simulink model "HR"  (R2022a)
settings: Solver=FixedStepDiscrete  StartTime=0.0  StopTime=0.04  FixedStep=0.04  RelTol=1e-3
PreLoadFcn:
  | listing = dir;
  | if (contains([listing .name], 'AGR')) && (contains([listing .name], 'MAP'))
  |     addpath('./AGR', './MAP');
  |     addpath( genpath('./MAP') );
  | elseif (contains([listing .name], 'HR.slx'))
  |     addpath('../AGR', '../MAP');
  |     addpath( genpath('../MAP') );
  | else
  | 
  | end
  | 
  | load('BusStructureHR.mat');
InitFcn:
  | listing = dir;
  | if (contains([listing .name], 'AGR')) && (contains([listing .name], 'MAP'))
  |     addpath('./AGR', './MAP');
  |     addpath( genpath('./MAP') );
  | elseif (contains([listing .name], 'HR.slx'))
  |     addpath('../AGR', '../MAP');
  |     addpath( genpath('../MAP') );
  | else
  | 
  | end
  | 
  | load('BusStructureHR.mat');
StartFcn:
  | listing = dir;
  | if (contains([listing .name], 'AGR')) && (contains([listing .name], 'MAP'))
  |     addpath('./AGR', './MAP');
  |     addpath( genpath('./MAP') );
  | elseif (contains([listing .name], 'HR.slx'))
  |     addpath('../AGR', '../MAP');
  |     addpath( genpath('../MAP') );
  | else
  | 
  | end
  | 
  | load('BusStructureHR.mat');
undefined symbols (not defined in the file or in its folder): HRDataTagWrap, HRElevationValid, HRImpactPointElevation, HRSelected, HRSelectedWraparound, HRTargetOffMap, HRTargetRangeEast, HRTargetRangeNorth, isFeasible, llh, ne, ned2ECEF, pECEF_ip, pECEF_ref, statusCode, targetLLH, targetNE
libraries: aerolibconvert2 x1
settings Model: Creator=ASCL  LastModifiedBy=ASCL
settings DataIOCC: SaveOutput=off  SignalLogging=off  DSMLogging=off  SaveTime=off  ReturnWorkspaceOutputs=off
settings OptimizationCC: BlockReduction=off  DefaultParameterBehavior=Inlined  UseDivisionForNetSlopeComputation=on  GainParamInheritBuiltInType=on  UseFloatMulNetSlope=on  ExpressionFolding=off  PassReuseOutputArgsAs=Individual arguments  ZeroExternalMemoryAtStartup=off  ZeroInternalMemoryAtStartup=off  EfficientFloat2IntCast=on  LifeSpan=inf  OptimizeBlockOrder=speed  DifferentSizesBufferReuse=on  EfficientTunableParamExpr=on
settings DebuggingCC: SignalInfNanChecking=warning  ReadBeforeWriteMsg=EnableAllAsWarning  WriteAfterWriteMsg=EnableAllAsError  WriteAfterReadMsg=EnableAllAsError  IntegerOverflowMsg=error  ParameterTunabilityLossMsg=error  UniqueDataStoreMsg=error  AssertControl=DisableAll  NonBusSignalsTreatedAsBus=error  SFInvalidInputDataAccessInChartInitDiag=error  SFTransitionOutsideNaturalParentDiag=error  SFUnreachableExecutionPathDiag=error  SFUndirectedBroadcastEventsDiag=error  IntegerSaturationMsg=error
settings HardwareCC: ProdBitPerPointer=32  ProdBitPerSizeT=32  ProdBitPerPtrDiffT=32  ProdLargestAtomicInteger=Long  ProdLargestAtomicFloat=Double  ProdEndianess=BigEndian  ProdWordSize=32  ProdLongLongMode=on  ProdHWDeviceType=Freescale->MPC83xx
settings ModelReferenceCC: ModelReferenceNumInstancesAllowed=Single
settings SFSimCC: SimCustomHeaderCode="#include \"MAP.h\""  SimUserSources=MAP.c  SimUserLibraries=WS2_32.LIB  CompileTimeRecursionLimit=0  EnableRuntimeRecursion=off  MATLABDynamicMemAlloc=off
settings RTWCC: SystemTargetFile=ert.tlc  TemplateMakefile=ert_default_tmf  GenerateReport=on  RTWUseSimCustomCode=on  CustomHeaderCode="#include \"MAP.h\""  CustomSource=MAP.c  CustomLibrary=WS2_32.LIB  BuildConfiguration=Faster Runs  IncludeHyperlinkInReport=on  LaunchReport=on  GenerateTraceInfo=on  GenerateTraceReport=on  GenerateTraceReportSl=on  GenerateTraceReportSf=on  GenerateTraceReportEml=on  GenerateCodeMetricsReport=on
settings CodeAppCC: ForceParamTrailComments=on  IgnoreCustomStorageClasses=off  OperatorAnnotations=on  SimulinkDataObjDesc=on  SFDataObjDesc=on  MATLABFcnDesc=on  InsertBlockDesc=on  StateflowObjectComments=on  MATLABSourceComments=on  EnableCustomComments=on  InlinedPrmAccess=Macros  ReqsInCode=on
settings ERTTargetCC: TargetLangStandard=C99 (ISO)  UtilityFuncGeneration=Shared location  GenerateSampleERTMain=on  IncludeMdlTerminateFcn=off  CombineSignalStateStructs=on  SuppressErrorStatus=on  SupportAbsoluteTime=off  SupportNonFinite=off  SupportComplex=off  SupportVariableSizeSignals=on  ParenthesesLevel=Standards  CastingMode=Standards  GenerateSharedConstants=off  InlinedParameterPlacement=NonHierarchical  ERTCustomFileTemplate=example_file_process.tlc  RateTransitionBlockCode=Function  PreserveIfCondition=on  ConvertIfToSwitch=off  EnableSignedLeftShifts=off  EnableSignedRightShifts=off

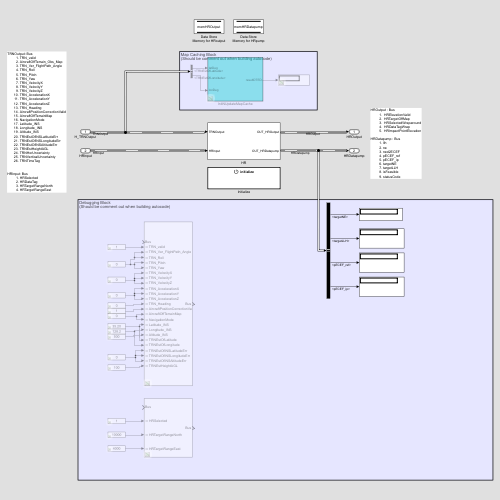
[thumbnail: Simulink's stored preview of the top-level diagram]
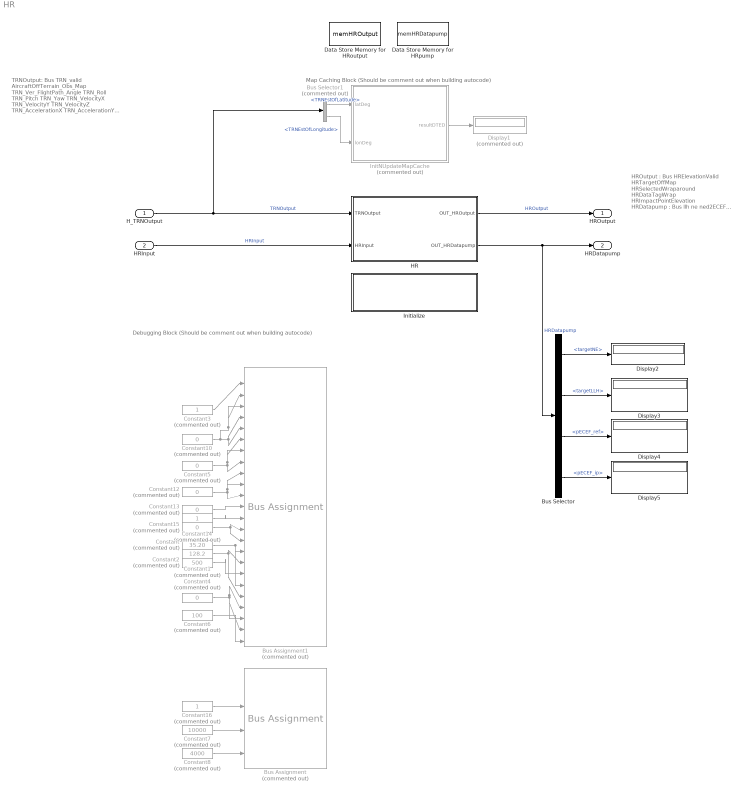
== system HR ==
  note: Debugging Block
      | (Should be comment out when building autocode)
  note: TRNOutput: Bus
      | TRN_valid
      | AircraftOffTerrain_Obs_Map
      | TRN_Ver_FlightPath_Angle
      | TRN_Roll
      | TRN_Pitch
      | TRN_Yaw
      | TRN_VelocityX
      | TRN_VelocityY
      | TRN_VelocityZ
      | TRN_AccelerationX
      | TRN_AccelerationY
      | TRN_AccelerationZ
      | TRN_Heading
      | AircraftPositionCorrectionValid
      | AircraftOffTerrainMap
      | NavigationMode
      | Latitude_INS
      | Longitude_INS
      | Altitude_INS
      | TRNEstOfINSLatitudeErr
      | TRNEstOfINSLongitudeErr
      | TRNEstOfINSAltitudeErr
      | TRNEstHeightAGL
      | TRNHorUncertainty
      | TRNVerticalUncertainty
      | TRNTimeTag
      |
      | HRInput: Bus
      | HRSelected
      | HRDataTag
      | HRTargetRangeNorth
      | HRTargetRangeEast
  note: HROutput : Bus
      | HRElevationValid
      | HRTargetOffMap
      | HRSelectedWraparound
      | HRDataTagWrap
      | HRImpactPointElevation
      |
      | HRDatapump : Bus
      | llh
      | ne
      | ned2ECEF
      | pECEF_ref
      | pECEF_ip
      | targetNE
      | targetLLH
      | isFeasible
      | statusCode
  note: Map Caching Block
      | (Should be comment out when building autocode)
  H_TRNOutput : Inport  OutDataTypeStr=Bus: TRNOutput  Interpolate=off  BusOutputAsStruct=on
  HRInput : Inport  Port=2  OutDataTypeStr=Bus: HRInput  Interpolate=off  BusOutputAsStruct=on
  Bus Assignment : BusAssignment  Commented=on  AssignedSignals=HRSelected,HRTargetRangeNorth,HRTargetRangeEast
  Bus Assignment1 : BusAssignment  Commented=on  AssignedSignals=TRN_valid,TRN_Ver_FlightPath_Angle,TRN_Roll,TRN_Pitch,TRN_Yaw,TRN_VelocityX,TRN_VelocityY,TRN_VelocityZ,TRN_AccelerationX,TRN_AccelerationY,TRN_AccelerationZ,TRN_Heading,AircraftPositionCorrectionValid,AircraftOffTerrainMap,NavigationMode,Latitude_INS,Longitude_INS,Altitude_INS,TRNEstOfLatitude,TRNEstOfLongitude,TRNEstOfINSLatitudeErr,TRNEstOfINSLongitudeErr,TRNEstOfINSAltitudeErr,TRNEstHeightAGL
  Bus Selector : BusSelector  OutputSignals=targetNE,targetLLH,pECEF_ref,pECEF_ip
  Bus Selector1 : BusSelector  Commented=on  OutputSignals=TRNEstOfLatitude,TRNEstOfLongitude
  Constant : Constant  Commented=on  Value=35.20
  Constant1 : Constant  Commented=on  Value=128.2
  Constant{4..5,10,12..13} (5 alike) : Constant  Commented=on  Value=0
  Constant14 : Constant  Commented=on  OutDataTypeStr=boolean
  Constant15 : Constant  Commented=on  Value=0  OutDataTypeStr=boolean
  Constant16 : Constant  Commented=on  OutDataTypeStr=boolean
  Constant2 : Constant  Commented=on  Value=500
  Constant3 : Constant  Commented=on  OutDataTypeStr=boolean
  Constant6 : Constant  Commented=on  Value=100  OutDataTypeStr=uint16
  Constant7 : Constant  Commented=on  Value=10000  OutDataTypeStr=double
  Constant8 : Constant  Commented=on  Value=4000  OutDataTypeStr=double
  Data Store Memory for HRoutput : DataStoreMemory  DataStoreName=memHROutput  ReadBeforeWriteMsg=warning  WriteAfterWriteMsg=warning  WriteAfterReadMsg=warning  VectorParams1D=off  ShowAdditionalParam=off  OutDataTypeStr=Bus: HROutput
  Data Store Memory for HRpump : DataStoreMemory  DataStoreName=memHRDatapump  ReadBeforeWriteMsg=warning  WriteAfterWriteMsg=warning  WriteAfterReadMsg=warning  VectorParams1D=off  ShowAdditionalParam=off  OutDataTypeStr=Bus: HRDatapump
  Display1 : Display  Commented=on
  Display{2..5} (4 alike) : Display
  HR : Subsystem
      mask init:
      | % latGPS = double(0);
      | % lonGPS = double(0);
      | % altGPS = double(0);
      | % velEGPS = double(0);
      | % velNGPS = double(0);
      | % velUGPS = double(0);
      | % notValidGPS = boolean(0);
      | % notAvaildINS = boolean(0);
      | % velUINS = double(0);
      | % velVINS = double(0);
      | % velWINS = double(0);
      | % rollINS = double(0);
      | % pitchINS = double(0);
      | % hgdINS = double(0);
      | % accXINS = double(0);
      | % accYINS = double(0);
      | % accZINS = double(0);
      | % activated = boolean(0);
      | % reactionT = uint16(0);
      | % pullUpG = uint16(0);
      | % rollRate = uint16(0);
      | % gOnsetRate = uint16(0);
      | % maxGamma = uint16(0);
      | % setWarnH = double(0);
      | % obsWarningTime = uint16(1);
      | % wiresWarningTime = uint16(1);
      | % latErrOfINS = double(0);
      | % lonErrOfINS = double(0);
      | % altErrorofINS = uint16(0);
      | % heightEstOfTRN = uint16(0);
      | % horUncertaintyOfTRN = double(0);
      | % verUncertaintyOfTRN = double(0);
  InitNUpdateMapCache : Subsystem  Commented=on  TreatAsAtomicUnit=on
  Initialize : Subsystem  TreatAsAtomicUnit=on
  HROutput : Outport  OutDataTypeStr=Bus: HROutput  VectorParamsAs1DForOutWhenUnconnected=off  BusOutputAsStruct=on
  HRDatapump : Outport  Port=2  OutDataTypeStr=Bus: HRDatapump  VectorParamsAs1DForOutWhenUnconnected=off  BusOutputAsStruct=on
  wires:
  Constant8/1 -> Bus Assignment/4
  Bus Selector/4 -> Display5/1  "<pECEF_ip>"
  Bus Selector/2 -> Display3/1  "<targetLLH>"
  H_TRNOutput/1 -> Bus Selector1/1, HR/1(TRNOutput)  "TRNOutput"
  Bus Selector/3 -> Display4/1  "<pECEF_ref>"
  Constant5/1 -> Bus Assignment1/7, Bus Assignment1/8, Bus Assignment1/9
  Constant6/1 -> Bus Assignment1/25
  Constant12/1 -> Bus Assignment1/10, Bus Assignment1/11, Bus Assignment1/12
  HRInput/1 -> HR/2(HRInput)  "HRInput"
  HR/2(OUT_HRDatapump) -> Bus Selector/1, HRDatapump/1  "HRDatapump"
  Constant16/1 -> Bus Assignment/2
  Constant10/1 -> Bus Assignment1/6, Bus Assignment1/5, Bus Assignment1/3, Bus Assignment1/4
  Constant13/1 -> Bus Assignment1/13
  Constant7/1 -> Bus Assignment/3
  Bus Selector/1 -> Display2/1  "<targetNE>"
  Constant2/1 -> Bus Assignment1/19
  Constant14/1 -> Bus Assignment1/14
  HR/1(OUT_HROutput) -> HROutput/1  "HROutput"
  Constant4/1 -> Bus Assignment1/22, Bus Assignment1/23, Bus Assignment1/24
  Constant1/1 -> Bus Assignment1/21, Bus Assignment1/18
  Constant/1 -> Bus Assignment1/20, Bus Assignment1/17
  Constant3/1 -> Bus Assignment1/2
  Constant15/1 -> Bus Assignment1/16, Bus Assignment1/15
  InitNUpdateMapCache/1(resultDTED) -> Display1/1
  Bus Selector1/1 -> InitNUpdateMapCache/1(latDeg)  "<TRNEstOfLatitude>"
  Bus Selector1/2 -> InitNUpdateMapCache/2(lonDeg)  "<TRNEstOfLongitude>"

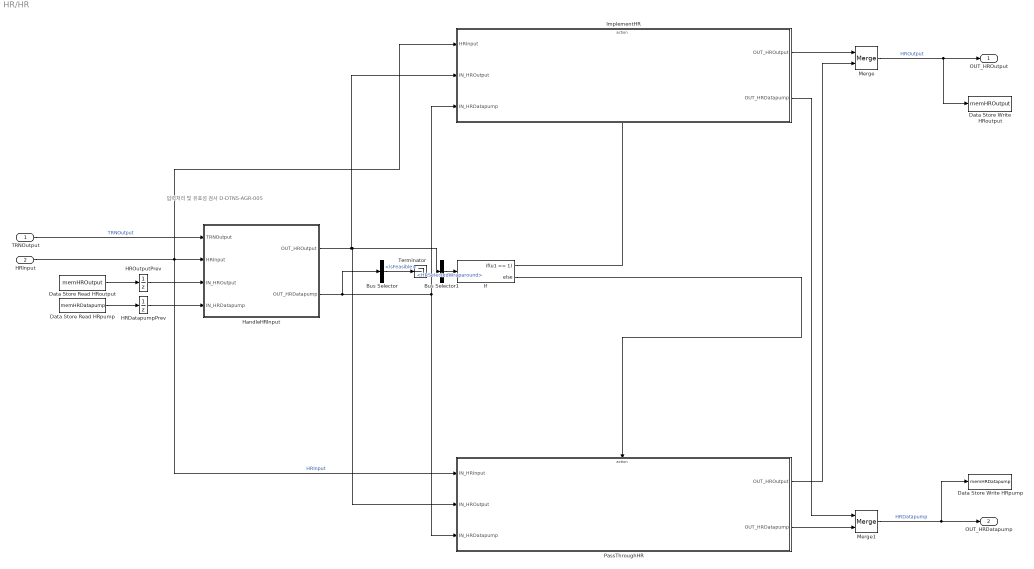
== system HR/HR ==
  note: 입력처리 및 유효성 검사 D-DTNS-AGR-005
  TRNOutput : Inport  OutDataTypeStr=Bus: TRNOutput
  HRInput : Inport  Port=2  OutDataTypeStr=Bus: HRInput
  Bus Selector : BusSelector  OutputSignals=isFeasible
  Bus Selector1 : BusSelector  OutputSignals=HRSelectedWraparound
  Data Store Read HRoutput : DataStoreRead  DataStoreName=memHROutput  IndexOptions=Index vector (dialog)  Indices=1  OutputSizes=1
  Data Store Read HRpump : DataStoreRead  DataStoreName=memHRDatapump  IndexOptions=Index vector (dialog)  Indices=1  OutputSizes=1
  Data Store Write HRoutput : DataStoreWrite  DataStoreName=memHROutput  IndexOptions=Index vector (dialog)  Indices=1  OutputSizes=1
  Data Store Write HRpump : DataStoreWrite  DataStoreName=memHRDatapump  IndexOptions=Index vector (dialog)  Indices=1  OutputSizes=1
  HRDatapumpPrev : UnitDelay  SampleTime=-1  HasFrameUpgradeWarning=on
  HROutputPrev : UnitDelay  SampleTime=-1  HasFrameUpgradeWarning=on
  HandleHRInput : Subsystem  TreatAsAtomicUnit=on
      settings: RTWSystemCode=Nonreusable function  RTWFcnNameOpts=Use subsystem name
  If : If  IfExpression=u1 == 1
  ImplementHR : Subsystem  TreatAsAtomicUnit=on
      settings: RTWSystemCode=Nonreusable function  RTWFcnNameOpts=Use subsystem name
  Merge : Merge
  Merge1 : Merge
  PassThroughHR : Subsystem  TreatAsAtomicUnit=on
      settings: RTWSystemCode=Nonreusable function  RTWFcnNameOpts=Use subsystem name
  Terminator : Terminator
  OUT_HROutput : Outport  OutDataTypeStr=Bus: HROutput  VectorParamsAs1DForOutWhenUnconnected=off
  OUT_HRDatapump : Outport  Port=2  OutDataTypeStr=Bus: HRDatapump  VectorParamsAs1DForOutWhenUnconnected=off
  wires:
  Merge/1 -> Data Store Write HRoutput/1, OUT_HROutput/1  "HROutput"
  Merge1/1 -> Data Store Write HRpump/1, OUT_HRDatapump/1  "HRDatapump"
  If/1 -> ImplementHR/Action
  If/2 -> PassThroughHR/Action
  Data Store Read HRoutput/1 -> HROutputPrev/1
  HRInput/1 -> ImplementHR/1(HRInput), PassThroughHR/1(IN_HRInput), HandleHRInput/2(HRInput)  "HRInput"
  Data Store Read HRpump/1 -> HRDatapumpPrev/1
  HandleHRInput/1(OUT_HROutput) -> Bus Selector1/1, PassThroughHR/2(IN_HROutput), ImplementHR/2(IN_HROutput)
  Bus Selector/1 -> Terminator/1  "<isFeasible>"
  HandleHRInput/2(OUT_HRDatapump) -> Bus Selector/1, PassThroughHR/3(IN_HRDatapump), ImplementHR/3(IN_HRDatapump)
  ImplementHR/1(OUT_HROutput) -> Merge/1
  PassThroughHR/2(OUT_HRDatapump) -> Merge1/2
  PassThroughHR/1(OUT_HROutput) -> Merge/2
  ImplementHR/2(OUT_HRDatapump) -> Merge1/1
  TRNOutput/1 -> HandleHRInput/1(TRNOutput)  "TRNOutput"
  HROutputPrev/1 -> HandleHRInput/3(IN_HROutput)
  HRDatapumpPrev/1 -> HandleHRInput/4(IN_HRDatapump)
  Bus Selector1/1 -> If/1  "<HRSelectedWraparound>"

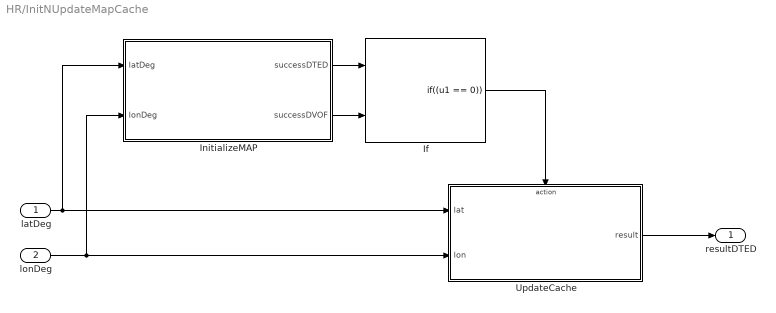
== system HR/InitNUpdateMapCache ==
  latDeg : Inport  OutDataTypeStr=double
  lonDeg : Inport  Port=2  OutDataTypeStr=double
  If : If  NumInputs=2  IfExpression=(u1 == 0)  ShowElse=off
  InitializeMAP : MATLAB Function  TreatAsAtomicUnit=on
  UpdateCache : Subsystem  TreatAsAtomicUnit=on
  resultDTED : Outport  VectorParamsAs1DForOutWhenUnconnected=off
  wires:
  UpdateCache/1(result) -> resultDTED/1
  InitializeMAP/1(successDTED) -> If/1
  latDeg/1 -> InitializeMAP/1(latDeg), UpdateCache/1(lat)
  InitializeMAP/2(successDVOF) -> If/2
  If/1 -> UpdateCache/Action
  lonDeg/1 -> InitializeMAP/2(lonDeg), UpdateCache/2(lon)

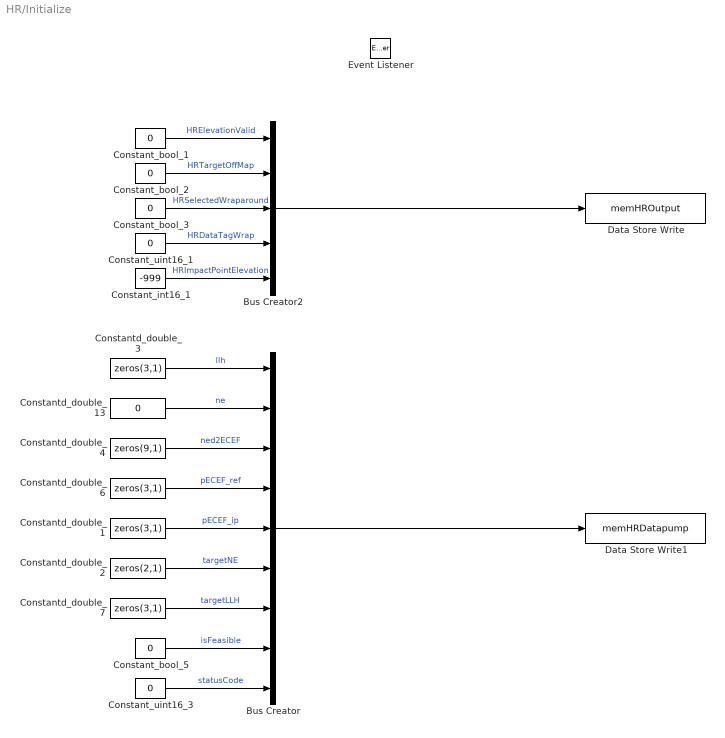
== system HR/Initialize ==
  Bus Creator : BusCreator  Inputs=9  OutDataTypeStr=Bus: HRDatapump  NonVirtualBus=on
  Bus Creator2 : BusCreator  Inputs=5  OutDataTypeStr=Bus: HROutput  NonVirtualBus=on
  Constant_bool_{1..3,5} (4 alike) : Constant  Value=0  OutDataTypeStr=boolean
  Constant_int16_1 : Constant  Value=-999  OutDataTypeStr=int16
  Constant_uint16_1 : Constant  Value=0  OutDataTypeStr=uint16
  Constant_uint16_3 : Constant  Value=0  OutDataTypeStr=uint16
  Constantd_double_{1,3,6..7} (4 alike) : Constant  Value=zeros(3,1)  OutDataTypeStr=double
  Constantd_double_13 : Constant  Value=0  OutDataTypeStr=double
  Constantd_double_2 : Constant  Value=zeros(2,1)  OutDataTypeStr=double
  Constantd_double_4 : Constant  Value=zeros(9,1)  OutDataTypeStr=double
  Data Store Write : DataStoreWrite  DataStoreName=memHROutput  IndexOptions=Index vector (dialog)  Indices=1  OutputSizes=1
  Data Store Write1 : DataStoreWrite  DataStoreName=memHRDatapump  IndexOptions=Index vector (dialog)  Indices=1  OutputSizes=1
  Event Listener : EventListener  DisableCoverage=on  EventName=reset
  wires:
  Bus Creator2/1 -> Data Store Write/1
  Constant_int16_1/1 -> Bus Creator2/5  "HRImpactPointElevation"
  Constant_uint16_1/1 -> Bus Creator2/4  "HRDataTagWrap"
  Constant_bool_1/1 -> Bus Creator2/1  "HRElevationValid"
  Constant_bool_2/1 -> Bus Creator2/2  "HRTargetOffMap"
  Constant_bool_3/1 -> Bus Creator2/3  "HRSelectedWraparound"
  Constantd_double_3/1 -> Bus Creator/1  "llh"
  Constantd_double_13/1 -> Bus Creator/2  "ne"
  Constantd_double_4/1 -> Bus Creator/3  "ned2ECEF"
  Constantd_double_6/1 -> Bus Creator/4  "pECEF_ref"
  Constantd_double_1/1 -> Bus Creator/5  "pECEF_ip"
  Constantd_double_2/1 -> Bus Creator/6  "targetNE"
  Constantd_double_7/1 -> Bus Creator/7  "targetLLH"
  Constant_bool_5/1 -> Bus Creator/8  "isFeasible"
  Constant_uint16_3/1 -> Bus Creator/9  "statusCode"
  Bus Creator/1 -> Data Store Write1/1

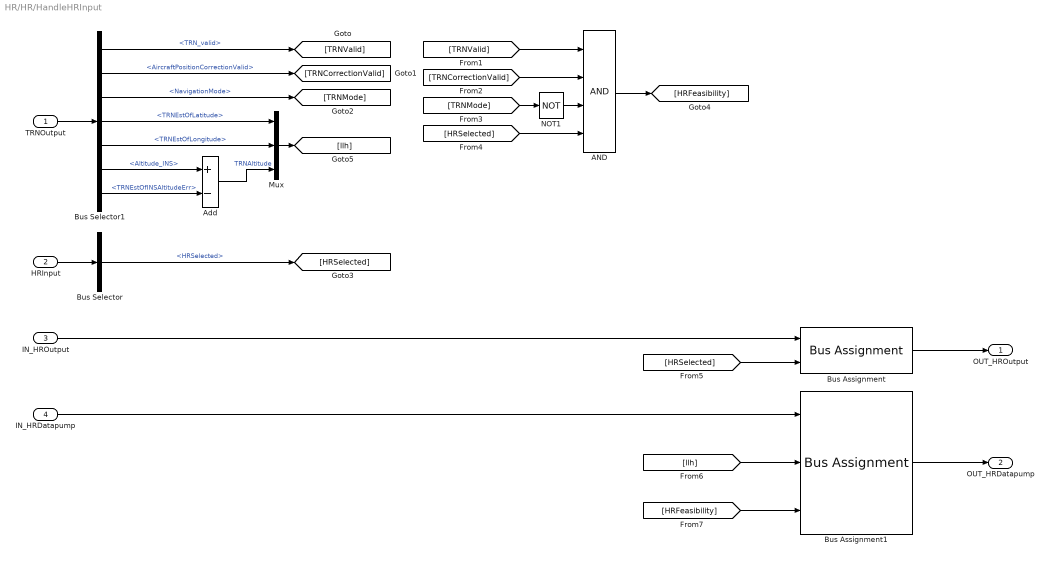
== system HR/HR/HandleHRInput ==
  TRNOutput : Inport  OutDataTypeStr=Bus: TRNOutput
  HRInput : Inport  Port=2  OutDataTypeStr=Bus: HRInput
  IN_HROutput : Inport  Port=3  OutDataTypeStr=Bus: HROutput
  IN_HRDatapump : Inport  Port=4  OutDataTypeStr=Bus: HRDatapump
  AND : Logic  Inputs=4  AllPortsSameDT=off  OutDataTypeStr=boolean
  Add : Sum  Inputs=+-
  Bus Assignment : BusAssignment  AssignedSignals=HRSelectedWraparound
  Bus Assignment1 : BusAssignment  AssignedSignals=llh,isFeasible
  Bus Selector : BusSelector  OutputSignals=HRSelected
  Bus Selector1 : BusSelector  OutputSignals=TRN_valid,AircraftPositionCorrectionValid,NavigationMode,TRNEstOfLatitude,TRNEstOfLongitude,Altitude_INS,TRNEstOfINSAltitudeErr
  Mux : Mux  Inputs=3
  NOT1 : Logic  Operator=NOT  IconShape=distinctive  AllPortsSameDT=off  OutDataTypeStr=boolean
  OUT_HROutput : Outport  OutDataTypeStr=Bus: HROutput  VectorParamsAs1DForOutWhenUnconnected=off
  OUT_HRDatapump : Outport  Port=2  OutDataTypeStr=Bus: HRDatapump  VectorParamsAs1DForOutWhenUnconnected=off
  wires:
  HRInput/1 -> Bus Selector/1
  IN_HROutput/1 -> Bus Assignment/1
  IN_HRDatapump/1 -> Bus Assignment1/1
  Bus Selector/1 -> [HRSelected]  "<HRSelected>"
  TRNOutput/1 -> Bus Selector1/1
  Bus Selector1/2 -> [TRNCorrectionValid]  "<AircraftPositionCorrectionValid>"
  Bus Selector1/1 -> [TRNValid]  "<TRN_valid>"
  Bus Selector1/3 -> [TRNMode]  "<NavigationMode>"
  [TRNValid] -> AND/1
  AND/1 -> [HRFeasibility]
  [TRNCorrectionValid] -> AND/2
  [HRSelected] -> AND/4
  NOT1/1 -> AND/3
  [TRNMode] -> NOT1/1
  Bus Assignment1/1 -> OUT_HRDatapump/1
  [llh] -> Bus Assignment1/2
  [HRFeasibility] -> Bus Assignment1/3
  Bus Selector1/4 -> Mux/1  "<TRNEstOfLatitude>"
  Mux/1 -> [llh]
  Bus Selector1/5 -> Mux/2  "<TRNEstOfLongitude>"
  Add/1 -> Mux/3  "TRNAltitude"
  Bus Selector1/7 -> Add/2  "<TRNEstOfINSAltitudeErr>"
  Bus Selector1/6 -> Add/1  "<Altitude_INS>"
  Bus Assignment/1 -> OUT_HROutput/1
  [HRSelected] -> Bus Assignment/2

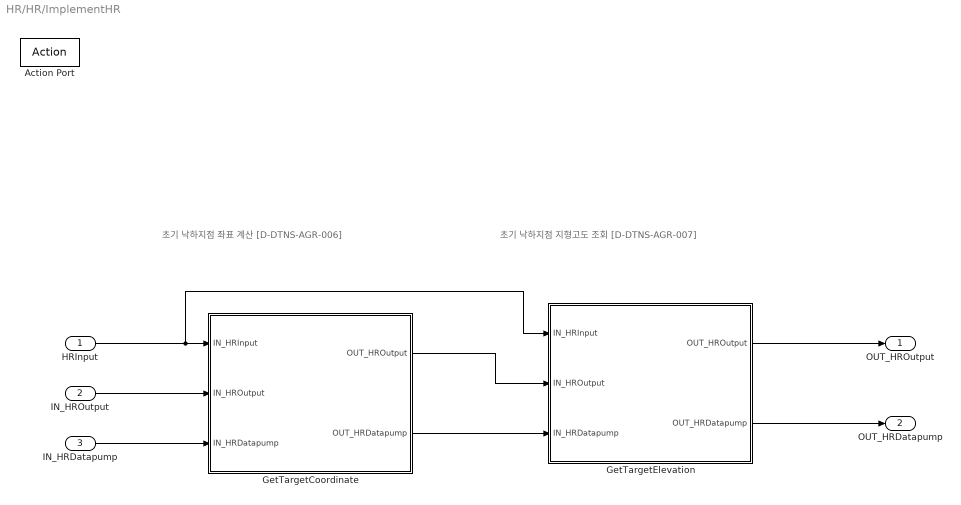
== system HR/HR/ImplementHR ==
  note: 초기 낙하지점 좌표 계산 [D-DTNS-AGR-006]
  note: 초기 낙하지점 지형고도 조회 [D-DTNS-AGR-007]
  HRInput : Inport  OutDataTypeStr=Bus: HRInput
  IN_HROutput : Inport  Port=2  OutDataTypeStr=Bus: HROutput
  IN_HRDatapump : Inport  Port=3  OutDataTypeStr=Bus: HRDatapump
  Action Port : ActionPort  ActionPortLabel=if(u1 == 1)
  GetTargetCoordinate : Subsystem  TreatAsAtomicUnit=on
      settings: RTWSystemCode=Nonreusable function  RTWFcnNameOpts=Use subsystem name
  GetTargetElevation : Subsystem  TreatAsAtomicUnit=on
      settings: RTWSystemCode=Nonreusable function  RTWFcnNameOpts=Use subsystem name
  OUT_HROutput : Outport  OutDataTypeStr=Bus: HROutput  VectorParamsAs1DForOutWhenUnconnected=off
  OUT_HRDatapump : Outport  Port=2  OutDataTypeStr=Bus: HRDatapump  VectorParamsAs1DForOutWhenUnconnected=off
  wires:
  GetTargetCoordinate/1(OUT_HROutput) -> GetTargetElevation/2(IN_HROutput)
  GetTargetCoordinate/2(OUT_HRDatapump) -> GetTargetElevation/3(IN_HRDatapump)
  IN_HRDatapump/1 -> GetTargetCoordinate/3(IN_HRDatapump)
  GetTargetElevation/1(OUT_HROutput) -> OUT_HROutput/1
  GetTargetElevation/2(OUT_HRDatapump) -> OUT_HRDatapump/1
  HRInput/1 -> GetTargetCoordinate/1(IN_HRInput), GetTargetElevation/1(IN_HRInput)
  IN_HROutput/1 -> GetTargetCoordinate/2(IN_HROutput)

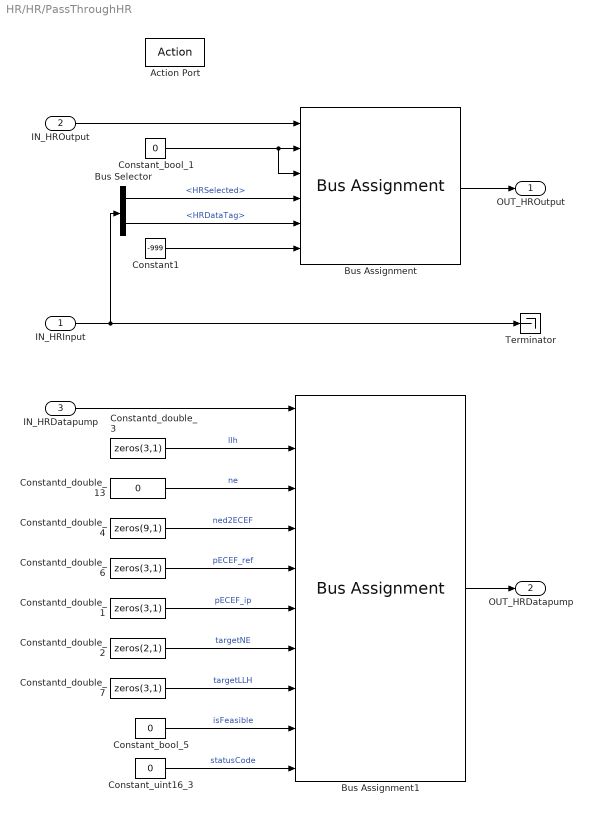
== system HR/HR/PassThroughHR ==
  IN_HRInput : Inport  OutDataTypeStr=Bus: HRInput
  IN_HROutput : Inport  Port=2  OutDataTypeStr=Bus: HROutput
  IN_HRDatapump : Inport  Port=3  OutDataTypeStr=Bus: HRDatapump
  Action Port : ActionPort  ActionPortLabel=else
  Bus Assignment : BusAssignment  AssignedSignals=HRElevationValid,HRTargetOffMap,HRSelectedWraparound,HRDataTagWrap,HRImpactPointElevation
  Bus Assignment1 : BusAssignment  AssignedSignals=llh,ne,ned2ECEF,pECEF_ref,pECEF_ip,targetNE,targetLLH,isFeasible,statusCode
  Bus Selector : BusSelector  OutputSignals=HRSelected,HRDataTag
  Constant1 : Constant  Value=-999  OutDataTypeStr=int16
  Constant_bool_1 : Constant  Value=0  OutDataTypeStr=boolean
  Constant_bool_5 : Constant  Value=0  OutDataTypeStr=boolean
  Constant_uint16_3 : Constant  Value=0  OutDataTypeStr=uint16
  Constantd_double_{1,3,6..7} (4 alike) : Constant  Value=zeros(3,1)  OutDataTypeStr=double
  Constantd_double_13 : Constant  Value=0  OutDataTypeStr=double
  Constantd_double_2 : Constant  Value=zeros(2,1)  OutDataTypeStr=double
  Constantd_double_4 : Constant  Value=zeros(9,1)  OutDataTypeStr=double
  Terminator : Terminator
  OUT_HROutput : Outport  OutDataTypeStr=Bus: HROutput  VectorParamsAs1DForOutWhenUnconnected=off
  OUT_HRDatapump : Outport  Port=2  OutDataTypeStr=Bus: HRDatapump  VectorParamsAs1DForOutWhenUnconnected=off
  wires:
  IN_HROutput/1 -> Bus Assignment/1
  Bus Assignment/1 -> OUT_HROutput/1
  IN_HRDatapump/1 -> Bus Assignment1/1
  IN_HRInput/1 -> Bus Selector/1, Terminator/1
  Bus Selector/2 -> Bus Assignment/5  "<HRDataTag>"
  Constant1/1 -> Bus Assignment/6
  Bus Selector/1 -> Bus Assignment/4  "<HRSelected>"
  Constant_bool_1/1 -> Bus Assignment/3, Bus Assignment/2
  Bus Assignment1/1 -> OUT_HRDatapump/1
  Constantd_double_13/1 -> Bus Assignment1/3  "ne"
  Constantd_double_1/1 -> Bus Assignment1/6  "pECEF_ip"
  Constantd_double_7/1 -> Bus Assignment1/8  "targetLLH"
  Constantd_double_2/1 -> Bus Assignment1/7  "targetNE"
  Constantd_double_6/1 -> Bus Assignment1/5  "pECEF_ref"
  Constantd_double_4/1 -> Bus Assignment1/4  "ned2ECEF"
  Constant_uint16_3/1 -> Bus Assignment1/10  "statusCode"
  Constant_bool_5/1 -> Bus Assignment1/9  "isFeasible"
  Constantd_double_3/1 -> Bus Assignment1/2  "llh"

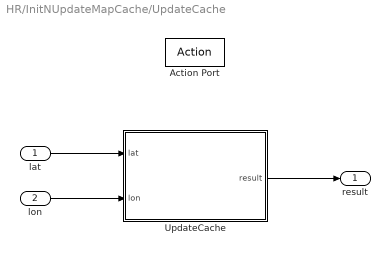
== system HR/InitNUpdateMapCache/UpdateCache ==
  lat : Inport
  lon : Inport  Port=2
  Action Port : ActionPort
  UpdateCache : MATLAB Function  TreatAsAtomicUnit=on
  result : Outport  VectorParamsAs1DForOutWhenUnconnected=off
  wires:
  UpdateCache/1(result) -> result/1
  lat/1 -> UpdateCache/1(lat)
  lon/1 -> UpdateCache/2(lon)

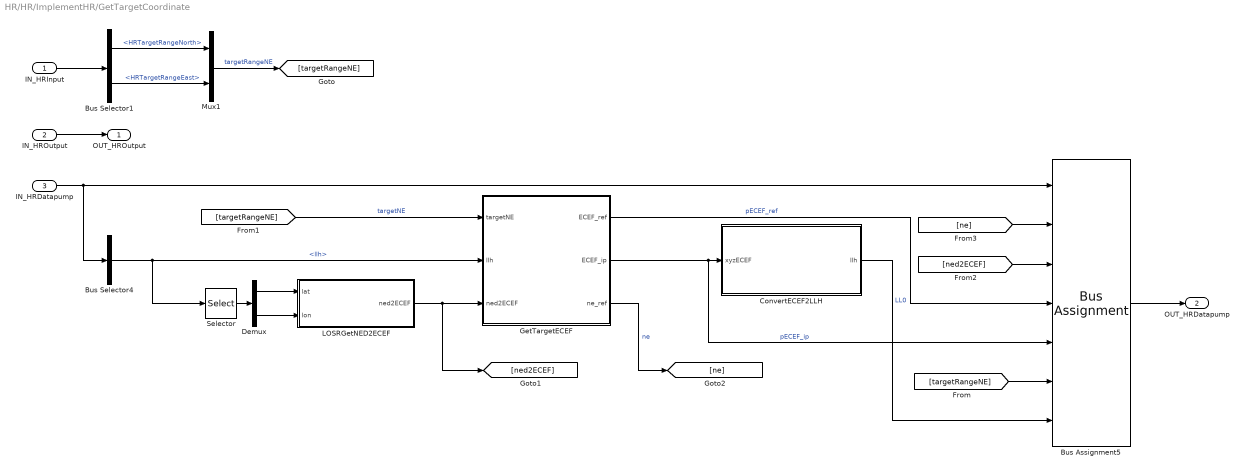
== system HR/HR/ImplementHR/GetTargetCoordinate ==
  IN_HRInput : Inport  OutDataTypeStr=Bus: HRInput
  IN_HROutput : Inport  Port=2  OutDataTypeStr=Bus: HROutput
  IN_HRDatapump : Inport  Port=3  OutDataTypeStr=Bus: HRDatapump
  Bus Assignment5 : BusAssignment  AssignedSignals=ne,ned2ECEF,pECEF_ref,pECEF_ip,targetNE,targetLLH
  Bus Selector1 : BusSelector  OutputSignals=HRTargetRangeNorth,HRTargetRangeEast
  Bus Selector4 : BusSelector  OutputSignals=llh
  ConvertECEF2LLH : MATLAB Function  TreatAsAtomicUnit=on
  Demux : Demux  Outputs=2
  GetTargetECEF : MATLAB Function  TreatAsAtomicUnit=on
  LOSRGetNED2ECEF : MATLAB Function  TreatAsAtomicUnit=on
  Mux1 : Mux  Inputs=2
  Selector : Selector  InputPortWidth=3  IndexOptions=Index vector (dialog)  Indices=[1 2]  OutputSizes=1
  OUT_HROutput : Outport  OutDataTypeStr=Bus: HROutput  VectorParamsAs1DForOutWhenUnconnected=off
  OUT_HRDatapump : Outport  Port=2  OutDataTypeStr=Bus: HRDatapump  VectorParamsAs1DForOutWhenUnconnected=off
  wires:
  IN_HRInput/1 -> Bus Selector1/1
  IN_HROutput/1 -> OUT_HROutput/1
  Bus Selector1/1 -> Mux1/1  "<HRTargetRangeNorth>"
  Bus Selector1/2 -> Mux1/2  "<HRTargetRangeEast>"
  Mux1/1 -> [targetRangeNE]  "targetRangeNE"
  IN_HRDatapump/1 -> Bus Selector4/1, Bus Assignment5/1
  Bus Assignment5/1 -> OUT_HRDatapump/1
  Bus Selector4/1 -> Selector/1, GetTargetECEF/2(llh)  "<llh>"
  GetTargetECEF/1(ECEF_ref) -> Bus Assignment5/4  "pECEF_ref"
  GetTargetECEF/2(ECEF_ip) -> Bus Assignment5/5, ConvertECEF2LLH/1(xyzECEF)  "pECEF_ip"
  [targetRangeNE] -> GetTargetECEF/1(targetNE)  "targetNE"
  [targetRangeNE] -> Bus Assignment5/6
  ConvertECEF2LLH/1(llh) -> Bus Assignment5/7  "LL0"
  Demux/1 -> LOSRGetNED2ECEF/1(lat)
  Demux/2 -> LOSRGetNED2ECEF/2(lon)
  Selector/1 -> Demux/1
  LOSRGetNED2ECEF/1(ned2ECEF) -> [ned2ECEF], GetTargetECEF/3(ned2ECEF)
  [ned2ECEF] -> Bus Assignment5/3
  GetTargetECEF/3(ne_ref) -> [ne]  "ne"
  [ne] -> Bus Assignment5/2

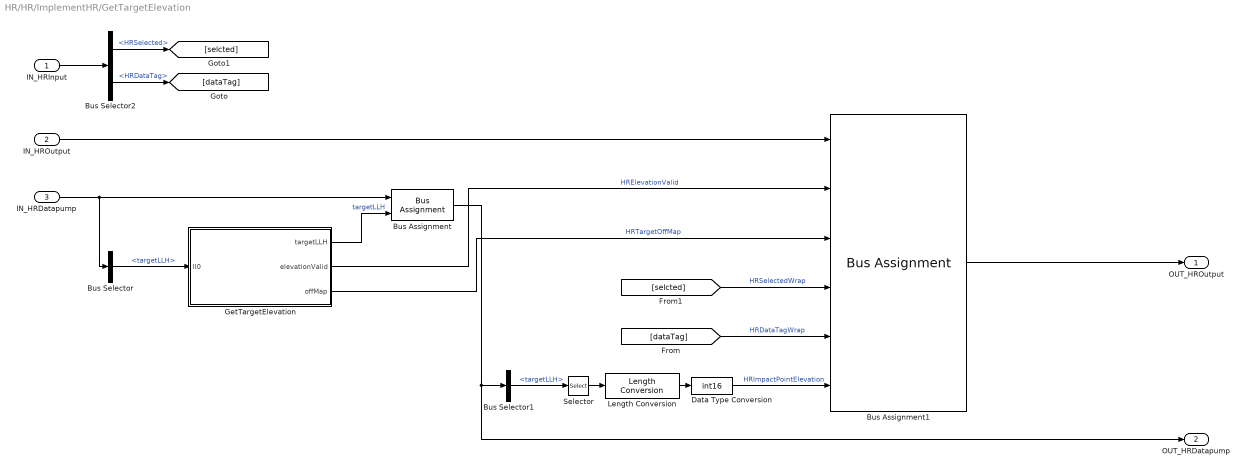
== system HR/HR/ImplementHR/GetTargetElevation ==
  IN_HRInput : Inport  OutDataTypeStr=Bus: HRInput
  IN_HROutput : Inport  Port=2  OutDataTypeStr=Bus: HROutput
  IN_HRDatapump : Inport  Port=3  OutDataTypeStr=Bus: HRDatapump
  Bus Assignment : BusAssignment  AssignedSignals=targetLLH
  Bus Assignment1 : BusAssignment  AssignedSignals=HRElevationValid,HRTargetOffMap,HRSelectedWraparound,HRDataTagWrap,HRImpactPointElevation
  Bus Selector : BusSelector  OutputSignals=targetLLH
  Bus Selector1 : BusSelector  OutputSignals=targetLLH
  Bus Selector2 : BusSelector  OutputSignals=HRSelected,HRDataTag
  Data Type Conversion : DataTypeConversion  OutDataTypeStr=int16  SaturateOnIntegerOverflow=off  RndMeth=Floor
  GetTargetElevation : MATLAB Function  TreatAsAtomicUnit=on
  Length Conversion : aerolibconvert2/Length Conversion  IU=m  OU=ft
  Selector : Selector  IndexMode=Zero-based  InputPortWidth=3  IndexOptions=Index vector (dialog)  Indices=2  OutputSizes=1
  OUT_HROutput : Outport  OutDataTypeStr=Bus: HROutput  VectorParamsAs1DForOutWhenUnconnected=off
  OUT_HRDatapump : Outport  Port=2  OutDataTypeStr=Bus: HRDatapump  VectorParamsAs1DForOutWhenUnconnected=off
  wires:
  IN_HRInput/1 -> Bus Selector2/1
  Bus Assignment/1 -> OUT_HRDatapump/1, Bus Selector1/1
  IN_HROutput/1 -> Bus Assignment1/1
  IN_HRDatapump/1 -> Bus Selector/1, Bus Assignment/1
  Bus Assignment1/1 -> OUT_HROutput/1
  Bus Selector1/1 -> Selector/1  "<targetLLH>"
  Bus Selector2/2 -> [dataTag]  "<HRDataTag>"
  Bus Selector/1 -> GetTargetElevation/1(ll0)  "<targetLLH>"
  GetTargetElevation/1(targetLLH) -> Bus Assignment/2  "targetLLH"
  Data Type Conversion/1 -> Bus Assignment1/6  "HRImpactPointElevation"
  [dataTag] -> Bus Assignment1/5  "HRDataTagWrap"
  Bus Selector2/1 -> [selcted]  "<HRSelected>"
  [selcted] -> Bus Assignment1/4  "HRSelectedWrap"
  GetTargetElevation/3(offMap) -> Bus Assignment1/3  "HRTargetOffMap"
  GetTargetElevation/2(elevationValid) -> Bus Assignment1/2  "HRElevationValid"
  Selector/1 -> Length Conversion/1
  Length Conversion/1 -> Data Type Conversion/1

== matlab function HR/ImplementHR/GetTargetElevation/GetTargetElevation ==
  data: targetLLH output; elevationValid output; ll0 input; offMap output
function [targetLLH, elevationValid, offMap] = GetTargetElevation(ll0)
%GetTargetElevation

% Initialize
targetLLH = zeros(3,1);
elevationValid = false;
offMap = false;

targetLLH = ll0;
EPSILON = 0.0001;

% Get Elevation
targetLLH(3) = coder.ceval('MAPGetTerrainHeight', ll0(1), ll0(2));

% Check Off Map
% if targetLLH(3) == -1.0
if abs(targetLLH(3)-(-1.0)) < EPSILON
    offMap = true;
    elevationValid = false;
    targetLLH(3) = -999;
else
    elevationValid = true;
end

== matlab function HR/ImplementHR/GetTargetCoordinate/ConvertECEF2LLH ==
  data: xyzECEF input; llh output
function llh  = ConvertECEF2LLH(xyzECEF)
%ConvertECEF2LLH
% Compute the {LLH} coordinates given {ECEF} coordinates
%
% == Inputs =========
% ecef              -  {ECEF} coordinates [m, m, m]
%
% == Outputs ========
% llh               - Corresponding Latitude, Longitude, Height [deg,deg,m]
%

% Initialize
llh = zeros(3,1);
lat     = 0.0;
lon     = 0.0;
h       = 0.0;

% WGS84 Parameters
r_e     = 6378137.0;            % major
f       = 1/298.257223563;      % (first) flattening
r_b     = r_e * (1-f);          % minor
e       = 0.08181919;           % Earth eccentricity
e2      = e*e;                  % Square of Earth eccentricity

% Rearrange
x       = xyzECEF(1);
y       = xyzECEF(2);
z       = xyzECEF(3);

% Longitude
lon = atan2d(y, x);

% Iteration for Latitude and Height [Bowring's method]

% Iteration parameters
eps     = 1;
tol     = 1e-12;

% side of triagle (hypotenuse: N+h, other side: z+N*e2*sind(lat) )
s       = sqrt(x^2 + y^2);

% Initial guesses
h   = 0.0;
N   = r_e;
lat = atand( z / (s * (1-e2*N/(N+h))) );

% Iteration terminates within 3~4 iterations.
count   = 0;

while (eps > tol) || (count > 10)
    lat0 = lat;

    % Recalculate
    h = s / cosd(lat) - N; 
    N   = r_e / sqrt(1-e2*(sind(lat))^2);
    lat = atand( z / (s * (1-e2*N/(N+h))) );

    % Update terminal condition parameters
    eps = abs(lat - lat0);
    count = count + 1;
end

llh = [lat; lon; h];

end

== matlab function HR/ImplementHR/GetTargetCoordinate/LOSRGetNED2ECEF ==
  data: lat input; ned2ECEF output; lon input
function ned2ECEF = LOSRGetNED2ECEF(lat, lon)
%LOSRGetNED2ECEF Compute transformation matrix from local NED to ECEF frame
% Input
% lat       : Current aircraft latitude [deg]
% lon       : Current aircraft longitude [deg]
% Output
% ned2ECEF  : Rotation matrix in single 1D array form
% *Note : (ECEF Vecotr) = (ned2ECEF) * (NED Vector) + (ECEF, Reference)

% Initialize
ned2ECEF = zeros(1,9);

% NED to ECEF Transformation Matrix
ned2ECEF(1,1) = -sind(lat)*cosd(lon);
ned2ECEF(1,2) = -sind(lon);
ned2ECEF(1,3) = -cosd(lat)*cosd(lon);

ned2ECEF(1,4) = -sind(lat)*sind(lon);
ned2ECEF(1,5) = cosd(lon);
ned2ECEF(1,6) = -cosd(lat)*sind(lon);

ned2ECEF(1,7) = cosd(lat);
ned2ECEF(1,8) = 0.0;
ned2ECEF(1,9) = -sind(lat);

end

== matlab function HR/ImplementHR/GetTargetCoordinate/GetTargetECEF ==
  data: ECEF_ref output; targetNE input; ECEF_ip output; llh input; ned2ECEF input; ne_ref output
function [ECEF_ref, ECEF_ip, ne_ref] = GetTargetECEF(targetNE, llh, ned2ECEF)
%GetTargetECEF

% Initialization
ECEF_ip = zeros(1,3);
ECEF_ref = zeros(1,3);
ne_ref = 0.0;

% Define constants
R_Ea            = 6378137.0;        % Earth semi-major axis [m]
e               = 0.08181919;       % Earth eccentricity

lat = llh(1);
lon = llh(2);
alt = llh(3);

% Prime vertical radius of curvature, N_{E} = ne
% (지구 횡 곡률반경)
ne_ref = R_Ea / sqrt(1 - e^2*(sind(lat))^2 );

% Calculate ECEF Coordinates of the current vehicle position as reference
ECEF_ref(1) = (ne_ref + alt) * cosd(lat) * cosd(lon);
ECEF_ref(2) = (ne_ref + alt) * cosd(lat) * sind(lon);
ECEF_ref(3) = (ne_ref * (1 - e^2) + alt) * sind(lat); 

% Calculate ECEF Coordinates of the impact point
% (target height is assumed to be zero)
pNED = [targetNE(1), targetNE(2), alt];

ECEF_ip(1) = ned2ECEF(1)*pNED(1) + ned2ECEF(2)*pNED(2) + ned2ECEF(3)*pNED(3) + ECEF_ref(1);
ECEF_ip(2) = ned2ECEF(4)*pNED(1) + ned2ECEF(5)*pNED(2) + ned2ECEF(6)*pNED(3) + ECEF_ref(2);
ECEF_ip(3) = ned2ECEF(7)*pNED(1) + ned2ECEF(8)*pNED(2) + ned2ECEF(9)*pNED(3) + ECEF_ref(3);

== matlab function HR/InitNUpdateMapCache/InitializeMAP ==
  data: successDTED output; successDVOF output; latDeg input; lonDeg input
function [successDTED, successDVOF] = InitializeMAP(latDeg, lonDeg)
%InitializeMAP

% Persistent variable
persistent firstRun
if isempty(firstRun)
    firstRun = true;
end

% Initialize output
flagDTED = int32(1);
flagDVOF = int32(1);
successDTED = int32(1);
successDVOF = int32(1);
hDEM = 0.0;

if firstRun
    % Path of DTED data
    pathDTED = 'C:\Users\ASCL\Documents\GitHub\DTNS\MAP\MAP_DB';

    % Length of DETD data path
    strLenDTED = int32(strlength(pathDTED));
    
    hDEM = coder.ceval('MAPGetTerrainHeight', latDeg, lonDeg);
    if IsNear(hDEM, -1.0)
        % Call [ InitialMap ] : 맵 폴더 위치 설정
        flagDTED = coder.ceval('InitialMap', pathDTED, strLenDTED );
        successDTED = flagDTED;
        if (~successDTED)
            firstRun = false;
        end
    else
        successDTED = int32(0);
        firstRun = false;       
    end
else
    successDTED = int32(0);
    successDVOF = int32(0);
end

== matlab function HR/InitNUpdateMapCache/UpdateCache/UpdateCache ==
  data: result output; lat input; lon input
function result = UpdateCache(lat, lon)
%UpdateCache

% Persistent variables
persistent latPrev lonPrev
if isempty(latPrev)
    latPrev = 0.0;
end
if isempty(lonPrev)
    lonPrev = 0.0;
end

% Initialize output
result = int32(1);

if ( abs(lat - latPrev) > 0.05 ) || ( abs(lon - lonPrev) > 0.05)
    result = coder.ceval('UpdateCache', lat, lon);
    latPrev = lat;
    lonPrev = lon;
else
    
end
